simulink model "Lab1"  (R2022a)
settings: Solver=VariableStepAuto  StartTime=0.0  StopTime=10  MaxStep=0.5  RelTol=1e-3
values from neighbouring files (symbols this model uses):
  gamma = 10    [code1.m]
  gamma_tild = gamma*k/k0    (= 20)    [code1.m]
  k = 2    [code1.m]
  k0 = 1    [code1.m]
libraries: simulink_extras x5
settings Model: Creator=fades  LastModifiedBy=fades

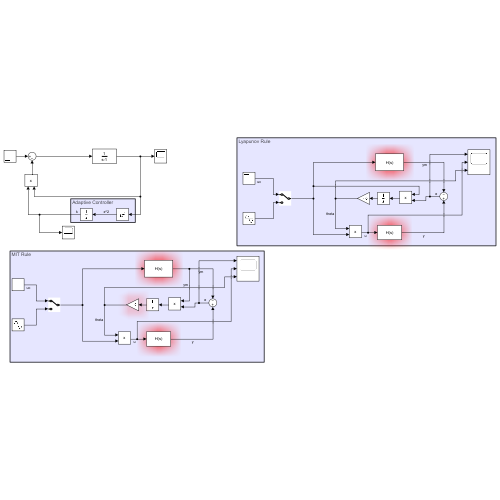
[thumbnail: Simulink's stored preview of the top-level diagram]
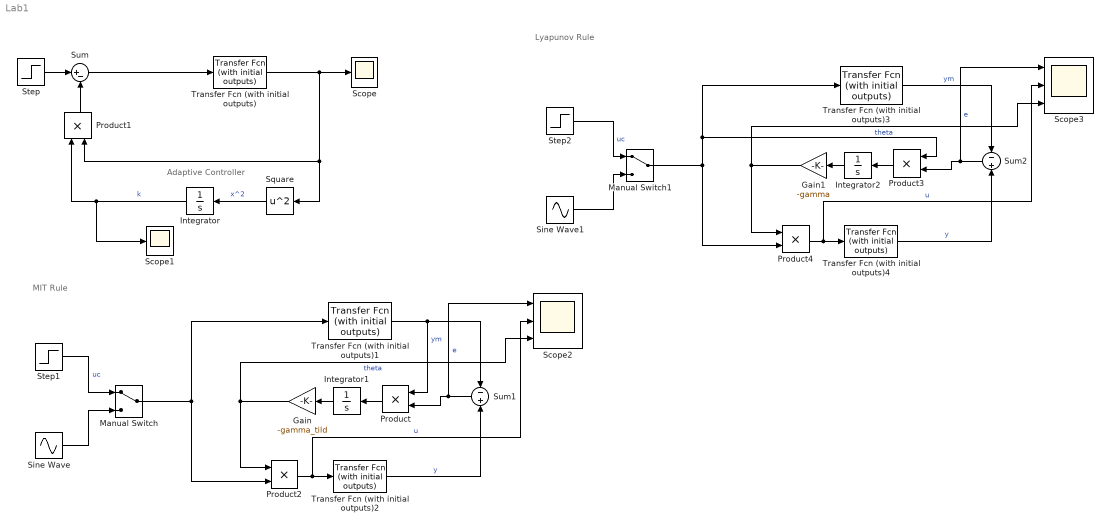
== system Lab1 ==
  note: Lyapunov Rule
  note: MIT Rule
  note: Adaptive Controller
  Gain : Gain  Gain=-gamma_tild
  Gain1 : Gain  Gain=-gamma
  Integrator : Integrator
  Integrator1 : Integrator
  Integrator2 : Integrator
  Manual Switch : ManualSwitch
  Manual Switch1 : ManualSwitch
  Product{,1..4} (5 alike) : Product
  Scope : Scope
  Scope1 : Scope
  Scope2 : Scope  NumInputPorts=3
  Scope3 : Scope  NumInputPorts=3
  Sine Wave : Sin  Frequency=0.15/pi  SampleTime=0
  Sine Wave1 : Sin  Frequency=0.15/pi  SampleTime=0
  Square : Math  Operator=square
  Step : Step  After=10  SampleTime=0
  Step1 : Step  After=-5  SampleTime=0
  Step2 : Step  After=-5  SampleTime=0
  Sum : Sum  Inputs=|+-
  Sum1 : Sum  Inputs=-+
  Sum2 : Sum  Inputs=-+
  Transfer Fcn (with initial outputs) : simulink_extras/Additional Linear/Transfer Fcn (with initial outputs)  N=[1]  D="[1  -1]"  Y0=0  U0=0
  Transfer Fcn (with initial outputs)1 : simulink_extras/Additional Linear/Transfer Fcn (with initial outputs)  N=[k0]  D="[1  1]"  Y0=0  U0=0
  Transfer Fcn (with initial outputs)2 : simulink_extras/Additional Linear/Transfer Fcn (with initial outputs)  N=[k]  D="[1  1]"  Y0=0  U0=0
  Transfer Fcn (with initial outputs)3 : simulink_extras/Additional Linear/Transfer Fcn (with initial outputs)  N=[k0]  D="[1  1]"  Y0=0  U0=0
  Transfer Fcn (with initial outputs)4 : simulink_extras/Additional Linear/Transfer Fcn (with initial outputs)  N=[k]  D="[1  1]"  Y0=0  U0=0
  wires:
  Transfer Fcn (with initial outputs)/1 -> Product1/2, Square/1, Scope/1
  Square/1 -> Integrator/1  "x^2"
  Product1/1 -> Sum/2
  Sum/1 -> Transfer Fcn (with initial outputs)/1
  Integrator/1 -> Scope1/1, Product1/1  "k"
  Step/1 -> Sum/1
  Transfer Fcn (with initial outputs)2/1 -> Sum1/2  "y"
  Transfer Fcn (with initial outputs)1/1 -> Product/1, Sum1/1  "ym"
  Sum1/1 -> Scope2/1, Product/2  "e"
  Product/1 -> Integrator1/1
  Integrator1/1 -> Gain/1
  Product2/1 -> Scope2/2, Transfer Fcn (with initial outputs)2/1  "u"
  Gain/1 -> Product2/1, Scope2/3  "theta"
  Manual Switch/1 -> Product2/2, Transfer Fcn (with initial outputs)1/1
  Step1/1 -> Manual Switch/1  "uc"
  Sine Wave/1 -> Manual Switch/2
  Sine Wave1/1 -> Manual Switch1/2
  Step2/1 -> Manual Switch1/1  "uc"
  Product3/1 -> Integrator2/1
  Gain1/1 -> Product4/1, Scope3/3  "theta"
  Transfer Fcn (with initial outputs)4/1 -> Sum2/2  "y"
  Integrator2/1 -> Gain1/1
  Manual Switch1/1 -> Product4/2, Product3/1, Transfer Fcn (with initial outputs)3/1
  Product4/1 -> Scope3/2, Transfer Fcn (with initial outputs)4/1  "u"
  Sum2/1 -> Scope3/1, Product3/2  "e"
  Transfer Fcn (with initial outputs)3/1 -> Sum2/1  "ym"
